simulink model "v3"  (R2024b)
settings: Solver=VariableStepAuto  StartTime=0.0  StopTime=Tsim  RelTol=1e-3
values from neighbouring files (symbols this model uses):
  a = am    (= 10)    [params_nonlinear_ref_model.m]
  am = 1/tauM    (= 10)    [params_nonlinear_ref_model.m]
  amplitude = 1    [params_nonlinear_ref_model.m]
  b = bm    (= 10)    [params_nonlinear_ref_model.m]
  BETA = BETA_m    (= 2)    [params_nonlinear_ref_model.m]    (also in test.m)
  BETA_m = 2    [params_nonlinear_ref_model.m]
  bias = 0    [params_nonlinear_ref_model.m]
  bm = K/tauM    (= 10)    [params_nonlinear_ref_model.m]
  epsilon = eps    [params_nonlinear_ref_model.m]
  IC_P = IC_Pm    (= 0)    [params_nonlinear_ref_model.m]
  IC_Pm = 0    [params_nonlinear_ref_model.m]
  period = 15    [params_nonlinear_ref_model.m]
  phase_delay = 0    [params_nonlinear_ref_model.m]
  pulse_width = 0.5    [params_nonlinear_ref_model.m]
  SAT_ACTIVE = 1    [params_nonlinear_ref_model.m]
  SIGNAL_NR = 2    [params_nonlinear_ref_model.m]
  w = 0    [params_nonlinear_ref_model.m]
  WEIGHT_UPDATE = 1    [params_nonlinear_ref_model.m]
  wm = 20    [params_nonlinear_ref_model.m]
settings Model: Creator=dalimwahby  LastModifiedBy=wahby
settings RTWCC: GPUComputeCapability=3.5

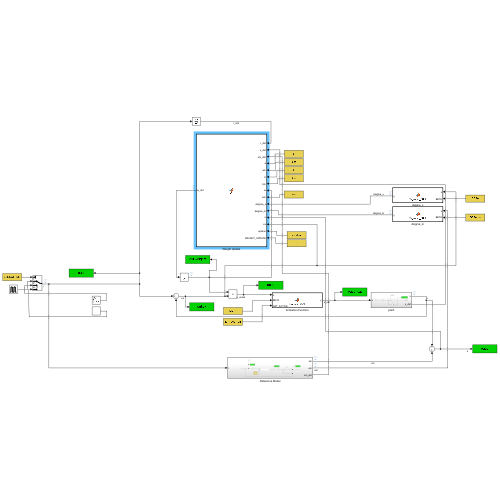
[thumbnail: Simulink's stored preview of the top-level diagram]
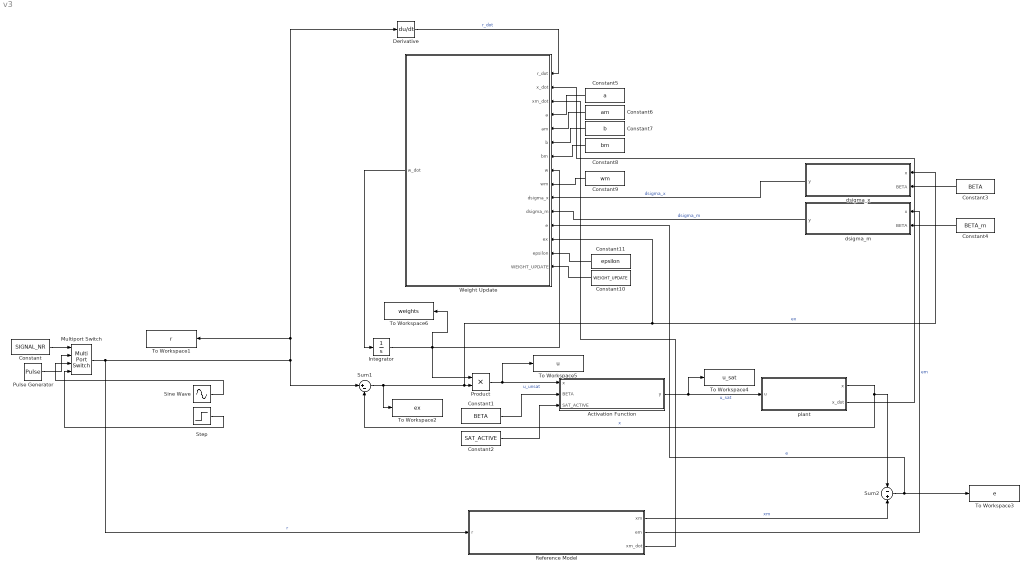
== system v3 ==
  Activation Function : MATLAB Function  TreatAsAtomicUnit=on
  Constant : Constant  Value=SIGNAL_NR
  Constant1 : Constant  Value=BETA
  Constant10 : Constant  Value=WEIGHT_UPDATE
  Constant11 : Constant  Value=epsilon
  Constant2 : Constant  Value=SAT_ACTIVE
  Constant3 : Constant  Value=BETA
  Constant4 : Constant  Value=BETA_m
  Constant5 : Constant  Value=a
  Constant6 : Constant  Value=am
  Constant7 : Constant  Value=b
  Constant8 : Constant  Value=bm
  Constant9 : Constant  Value=wm
  Derivative : Derivative
  Integrator : Integrator  InitialCondition=w
  Multiport Switch : MultiPortSwitch  SaturateOnIntegerOverflow=off  InputSameDT=off
  Product : Product
  Pulse Generator : DiscretePulseGenerator  PulseType=Time based  Amplitude=amplitude  Period=period  PulseWidth=pulse_width*100  PhaseDelay=phase_delay
  Reference Model : Subsystem
  Sine Wave : Sin  Amplitude=amplitude  Bias=bias  SampleTime=0
  Step : Step  Time=phase_delay  After=amplitude  SampleTime=0
  Sum1 : Sum  Inputs=|+-
  Sum2 : Sum  Inputs=-+
  To Workspace1 : ToWorkspace  VariableName=r  SaveFormat=Timeseries  SampleTime=-1
  To Workspace2 : ToWorkspace  VariableName=ex  SaveFormat=Timeseries  SampleTime=-1
  To Workspace3 : ToWorkspace  VariableName=e  SaveFormat=Timeseries  SampleTime=-1
  To Workspace4 : ToWorkspace  VariableName=u_sat  SaveFormat=Timeseries  SampleTime=-1
  To Workspace5 : ToWorkspace  VariableName=u  SaveFormat=Timeseries  SampleTime=-1
  To Workspace6 : ToWorkspace  VariableName=weights  SaveFormat=Timeseries  SampleTime=-1
  Weight Update : MATLAB Function  TreatAsAtomicUnit=on
  dsigma_m : MATLAB Function  TreatAsAtomicUnit=on
  dsigma_x : MATLAB Function  TreatAsAtomicUnit=on
  plant : Subsystem
  wires:
  Sum1/1 -> Weight Update/13(ex), dsigma_x/1(x), Product/2, To Workspace2/1  "ex"
  plant/1(x) -> Sum2/1, Sum1/2  "x"
  Constant/1 -> Multiport Switch/1
  Product/1 -> To Workspace5/1, Activation Function/1(x)  "u_unsat"
  Activation Function/1(y) -> plant/1(u), To Workspace4/1  "u_sat"
  Constant2/1 -> Activation Function/3(SAT_ACTIVE)
  Multiport Switch/1 -> Derivative/1, To Workspace1/1, Sum1/1, Reference Model/1(r)  "r"
  Sum2/1 -> To Workspace3/1, Weight Update/12(e)  "e"
  Constant1/1 -> Activation Function/2(BETA)
  Pulse Generator/1 -> Multiport Switch/2
  Sine Wave/1 -> Multiport Switch/3
  Reference Model/1(xm) -> Sum2/2  "xm"
  Step/1 -> Multiport Switch/4
  Integrator/1 -> Product/1, To Workspace6/1, Weight Update/8(w)
  Weight Update/1(w_dot) -> Integrator/1
  dsigma_x/1(y) -> Weight Update/10(dsigma_x)  "dsigma_x"
  dsigma_m/1(y) -> Weight Update/11(dsigma_m)  "dsigma_m"
  Constant4/1 -> dsigma_m/2(BETA)
  Constant3/1 -> dsigma_x/2(BETA)
  Reference Model/2(em) -> dsigma_m/1(x)  "em"
  plant/2(x_dot) -> Weight Update/2(x_dot)
  Reference Model/3(xm_dot) -> Weight Update/3(xm_dot)
  Constant5/1 -> Weight Update/4(a)
  Constant6/1 -> Weight Update/5(am)
  Constant7/1 -> Weight Update/6(b)
  Constant8/1 -> Weight Update/7(bm)
  Constant9/1 -> Weight Update/9(wm)
  Constant10/1 -> Weight Update/15(WEIGHT_UPDATE)
  Constant11/1 -> Weight Update/14(epsilon)
  Derivative/1 -> Weight Update/1(r_dot)  "r_dot"

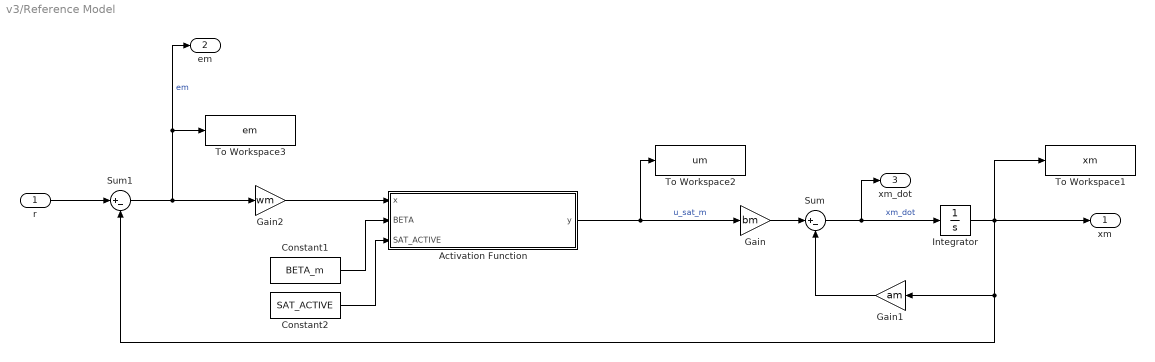
== system v3/Reference Model ==
  r : Inport
  Activation Function : MATLAB Function  TreatAsAtomicUnit=on
  Constant1 : Constant  Value=BETA_m
  Constant2 : Constant  Value=SAT_ACTIVE
  Gain : Gain  Gain=bm
  Gain1 : Gain  Gain=am
  Gain2 : Gain  Gain=wm
  Integrator : Integrator  InitialCondition=IC_Pm
  Sum : Sum  Inputs=|+-
  Sum1 : Sum  Inputs=|+-
  To Workspace1 : ToWorkspace  VariableName=xm  SaveFormat=Timeseries  SampleTime=-1
  To Workspace2 : ToWorkspace  VariableName=um  SaveFormat=Timeseries  SampleTime=-1
  To Workspace3 : ToWorkspace  VariableName=em  SaveFormat=Timeseries  SampleTime=-1
  xm : Outport
  em : Outport  Port=2
  xm_dot : Outport  Port=3
  wires:
  Constant2/1 -> Activation Function/3(SAT_ACTIVE)
  Sum/1 -> xm_dot/1, Integrator/1  "xm_dot"
  Constant1/1 -> Activation Function/2(BETA)
  Gain1/1 -> Sum/2
  Activation Function/1(y) -> To Workspace2/1, Gain/1  "u_sat_m"
  Integrator/1 -> Sum1/2, Gain1/1, xm/1, To Workspace1/1
  Gain/1 -> Sum/1
  Gain2/1 -> Activation Function/1(x)
  r/1 -> Sum1/1
  Sum1/1 -> em/1, To Workspace3/1, Gain2/1  "em"

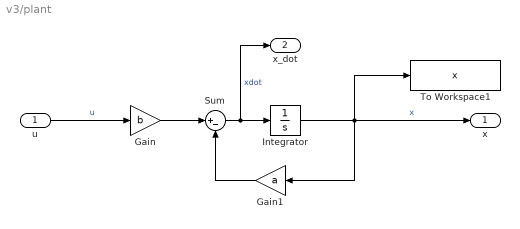
== system v3/plant ==
  u : Inport
  Gain : Gain  Gain=b
  Gain1 : Gain  Gain=a
  Integrator : Integrator  InitialCondition=IC_P
  Sum : Sum  Inputs=|+-
  To Workspace1 : ToWorkspace  VariableName=x  SaveFormat=Timeseries  SampleTime=-1
  x : Outport
  x_dot : Outport  Port=2
  wires:
  u/1 -> Gain/1  "u"
  Sum/1 -> x_dot/1, Integrator/1  "xdot"
  Integrator/1 -> Gain1/1, x/1, To Workspace1/1  "x"
  Gain1/1 -> Sum/2
  Gain/1 -> Sum/1

== matlab function v3/Activation Function ==
  data: x input; y output; BETA input; SAT_ACTIVE input
function y = Sigmoid_SAT(x, BETA, SAT_ACTIVE)
    if SAT_ACTIVE==1
        y = (2*(1-exp(-BETA.*x)))./(BETA*(1+exp(-BETA.*x)));
    else
        y = x;
    end
end

== matlab function v3/Reference Model/Activation Function ==
  data: x input; y output; BETA input; SAT_ACTIVE input
function y = Sigmoid_SAT(x, BETA, SAT_ACTIVE)
    if SAT_ACTIVE==1
        y = (2*(1-exp(-BETA.*x)))./(BETA*(1+exp(-BETA.*x)));
    else
        y = x;
    end
end

== matlab function v3/Weight Update ==
  data: r_dot input; x_dot input; xm_dot input; a input; am input; b input; bm input; w input; wm input; dsigma_x input; dsigma_m input; e input; ex input; epsilon input; WEIGHT_UPDATE input; w_dot output
function w_dot = fcn(r_dot, x_dot, xm_dot, a, am, b, bm, w, wm, dsigma_x, dsigma_m, e, ex, epsilon, WEIGHT_UPDATE)
if WEIGHT_UPDATE==0
    w_dot = 0;
else
    if (abs(ex)<epsilon)
        w_dot=0;
    else
        
        w_dot = ((1/(ex*b*dsigma_x))*(e + (a-am)*x_dot + bm*dsigma_m*wm*(r_dot-xm_dot))) - (w/ex)*(r_dot-x_dot);
        %w_dot = (1/(ex*b*dsigma_x))*(e + (a-am)*x_dot + bm*dsigma_m*wm*em_dot) - (w/ex)*(ex_dot);
    end
end

== matlab function v3/dsigma_x ==
  data: x input; y output; BETA input
function y = Sigmoid_SAT(x, BETA)

y = (2*(1-exp(-BETA.*x)))./(BETA*(1+exp(-BETA.*x)));
end

== matlab function v3/dsigma_m ==
  data: x input; y output; BETA input
function y = Sigmoid_SAT(x, BETA)

y = (2*(1-exp(-BETA.*x)))./(BETA*(1+exp(-BETA.*x)));
end
